simulink model "attitude_control"  (R2018a)
settings: Solver=VariableStepAuto  StartTime=0.0  StopTime=20  RelTol=1e-3
undefined symbols (not defined in the file): drone, matrix_A, matrix_B, matrix_C, matrix_D, obs_L, reg_K, simulation_sampling_ts
libraries: simulink x1
settings Model: Creator=ros  LastModifiedBy=ros

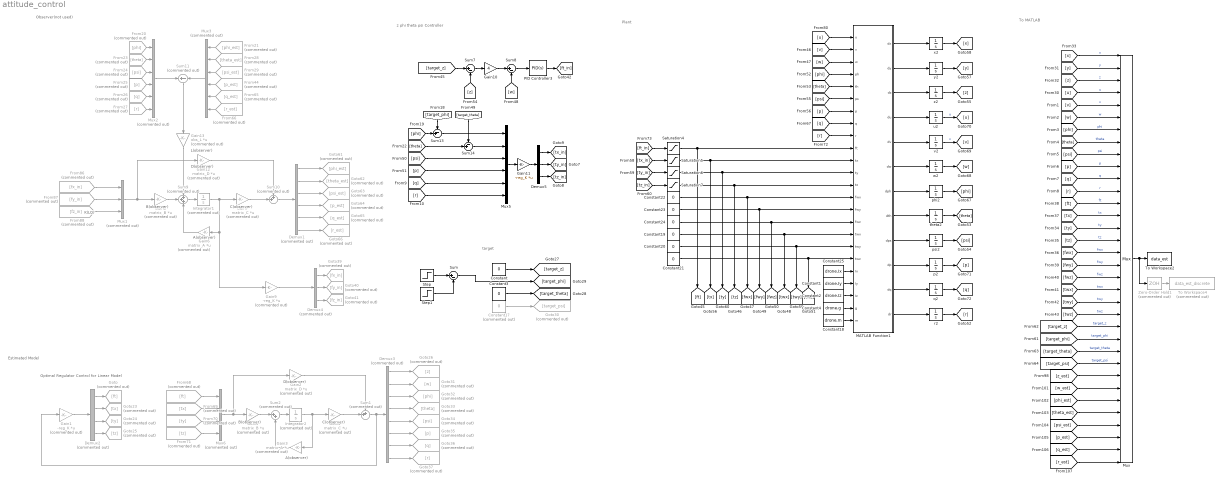
== system attitude_control ==
  note: B(observer)
  note: C(observer)
  note: A(observer)
  note: D(observer)
  note: L(observer)
  note: Optimal Regulator Control for Linear Model
  note: D(observer)
  note: C(observer)
  note: A(observer)
  note: B(observer)
  note: K(LQ)
  note: Plant
  note: To MATLAB
  note: target
  note: Estimated Model
  note: Observer(not used)
  note: z phi theta psi Controller
  Constant{,3,19..24} (8 alike) : Constant  Value=0
  Constant1 : Constant  Value=drone.Iy
  Constant17 : Constant  Commented=on  Value=0
  Constant18 : Constant  Value=drone.m
  Constant2 : Constant  Value=drone.Iz
  Constant25 : Constant  Value=drone.Ix
  Constant4 : Constant  Value=drone.g
  Demux1 : Demux  Commented=on  Outputs=6
  Demux2 : Demux  Commented=on
  Demux3 : Demux  Commented=on  Outputs=8
  Demux4 : Demux  Commented=on  Outputs=3
  Demux5 : Demux  Outputs=3
  From20 : From  Commented=on  GotoTag=phi
  From21 : From  Commented=on  GotoTag=phi_est
  From23 : From  Commented=on  GotoTag=theta
  From24 : From  Commented=on  GotoTag=psi
  From25 : From  Commented=on  GotoTag=p
  From26 : From  Commented=on  GotoTag=q
  From27 : From  Commented=on  GotoTag=r
  From28 : From  Commented=on  GotoTag=theta_est
  From29 : From  Commented=on  GotoTag=psi_est
  From44 : From  Commented=on  GotoTag=p_est
  From65 : From  Commented=on  GotoTag=q_est
  From66 : From  Commented=on  GotoTag=r_est
  From68 : From  Commented=on  GotoTag=ft
  From69 : From  Commented=on  GotoTag=tx
  From70 : From  Commented=on  GotoTag=ty
  From71 : From  Commented=on  GotoTag=tz
  From86 : From  Commented=on  GotoTag=fx_in
  From87 : From  Commented=on  GotoTag=fy_in
  From88 : From  Commented=on  GotoTag=fz_in
  Gain1 : Gain  Commented=on  Gain=-reg_K  Multiplication=Matrix(K*u)
  Gain10 : Gain  Gain=4
  Gain11 : Gain  Gain=-reg_K  Multiplication=Matrix(K*u)
  Gain12 : Gain  Commented=on  Gain=matrix_D  Multiplication=Matrix(K*u)
  Gain13 : Gain  Commented=on  Gain=obs_L  Multiplication=Matrix(K*u)
  Gain2 : Gain  Commented=on  Gain=matrix_D  Multiplication=Matrix(K*u)
  Gain3 : Gain  Commented=on  Gain=matrix_A  Multiplication=Matrix(K*u)
  Gain4 : Gain  Commented=on  Gain=matrix_C  Multiplication=Matrix(K*u)
  Gain5 : Gain  Commented=on  Gain=matrix_B  Multiplication=Matrix(K*u)
  Gain6 : Gain  Commented=on  Gain=matrix_A  Multiplication=Matrix(K*u)
  Gain7 : Gain  Commented=on  Gain=matrix_C  Multiplication=Matrix(K*u)
  Gain8 : Gain  Commented=on  Gain=matrix_B  Multiplication=Matrix(K*u)
  Gain9 : Gain  Commented=on  Gain=-reg_K  Multiplication=Matrix(K*u)
  Goto : Goto  Commented=on  GotoTag=ft
  Goto23 : Goto  Commented=on  GotoTag=tx
  Goto24 : Goto  Commented=on  GotoTag=ty
  Goto25 : Goto  Commented=on  GotoTag=tz
  Goto26 : Goto  Commented=on  GotoTag=z
  Goto30 : Goto  Commented=on  GotoTag=target_psi
  Goto31 : Goto  Commented=on  GotoTag=w
  Goto32 : Goto  Commented=on  GotoTag=phi
  Goto33 : Goto  Commented=on  GotoTag=theta
  Goto34 : Goto  Commented=on  GotoTag=psi
  Goto35 : Goto  Commented=on  GotoTag=p
  Goto36 : Goto  Commented=on  GotoTag=q
  Goto37 : Goto  Commented=on  GotoTag=r
  Goto39 : Goto  Commented=on  GotoTag=fx_in
  Goto40 : Goto  Commented=on  GotoTag=fy_in
  Goto41 : Goto  Commented=on  GotoTag=fz_in
  Goto61 : Goto  Commented=on  GotoTag=phi_est
  Goto62 : Goto  Commented=on  GotoTag=theta_est
  Goto63 : Goto  Commented=on  GotoTag=psi_est
  Goto64 : Goto  Commented=on  GotoTag=p_est
  Goto65 : Goto  Commented=on  GotoTag=q_est
  Goto66 : Goto  Commented=on  GotoTag=r_est
  Integrator1 : Integrator  Commented=on  InitialCondition=[0 0 0 0 0 0 0 0]
  Integrator2 : Integrator  Commented=on  InitialCondition=[-5 0 0 0 0 0 0 0]
  MATLAB Function1 : MATLAB Function  TreatAsAtomicUnit=on
  Mux : Mux  Inputs=34
      settings: DisplayOption=signals
  Mux1 : Mux  Commented=on  Inputs=3
  Mux2 : Mux  Commented=on  Inputs=6
  Mux3 : Mux  Commented=on  Inputs=6
  Mux5 : Mux  Inputs=6
  Mux6 : Mux  Commented=on
  PID Controller3 : simulink/Continuous/PID Controller  Controller=PID  TimeDomain=Continuous-time  SampleTime=-1  IntegratorMethod=Forward Euler  FilterMethod=Forward Euler  Form=Parallel  UseFilter=on  ControllerParametersSource=internal  P=7  I=6  D=0.7  N=100  InitialConditionSource=internal  InitialConditionForIntegrator=0  InitialConditionForFilter=0  ExternalReset=none  LimitOutput=off  UpperSaturationLimit=inf  LowerSaturationLimit=-inf  LinearizeAsGain=on  AntiWindupMode=none  Kb=1  TrackingMode=off  Kt=1  PParamMin=[]  PParamMax=[]  IParamMin=[]  IParamMax=[]  DParamMin=[]  DParamMax=[]  NParamMin=[]  NParamMax=[]  KbParamMin=[]  KbParamMax=[]  KtParamMin=[]  KtParamMax=[]  POutMin=[]  POutMax=[]  IOutMin=[]  IOutMax=[]  DOutMin=[]  DOutMax=[]  NOutMin=[]  NOutMax=[]  KbOutMin=[]  KbOutMax=[]  KtOutMin=[]  KtOutMax=[]  IntegratorOutMin=[]  IntegratorOutMax=[]  FilterOutMin=[]  FilterOutMax=[]  SumOutMin=[]  SumOutMax=[]  SumI1OutMin=[]  SumI1OutMax=[]  SumI2OutMin=[]  SumI2OutMax=[]  SumI3OutMin=[]  SumI3OutMax=[]  SumDOutMin=[]  SumDOutMax=[]  SaturationOutMin=[]  SaturationOutMax=[]  IntegratorContinuousStateAttributes=''  IntegratorStateMustResolveToSignalObject=off  IntegratorRTWStateStorageClass=Auto  FilterContinuousStateAttributes=''  FilterStateMustResolveToSignalObject=off  FilterRTWStateStorageClass=Auto  DifferentiatorICPrevScaledInput=0  DifferentiatorOutMin=[]  DifferentiatorOutMax=[]  FilterDiffOutCoefMin=[]  FilterDiffOutCoefMax=[]  SumDenOutMin=[]  SumDenOutMax=[]  SumNumOutMin=[]  SumNumOutMax=[]  ReciprocalOutMin=[]  ReciprocalOutMax=[]  DivideOutMin=[]  DivideOutMax=[]  TunerSelectOption=Transfer Function Based (PID Tuner App)
  Saturation{4..7} (4 alike) : Saturate  UpperLimit=30  LowerLimit=-100
  Step : Step  After=5*pi/180  SampleTime=0
  Step1 : Step  Time=6  After=5*pi/180  SampleTime=0
  Sum : Sum  Inputs=|+-
  Sum1 : Sum  Commented=on  Inputs=++|
  Sum10 : Sum  Commented=on  Inputs=++|
  Sum11 : Sum  Commented=on  Inputs=+-
  Sum13 : Sum  Inputs=-+|
  Sum14 : Sum  Inputs=-+|
  Sum2 : Sum  Commented=on  Inputs=|++
  Sum7 : Sum  Inputs=|+-
  Sum8 : Sum  Inputs=|+-
  Sum9 : Sum  Commented=on  Inputs=+++
  To Workspace2 : ToWorkspace  VariableName=data_est  SaveFormat=Timeseries  SampleTime=-1
  To Workspace4 : ToWorkspace  Commented=on  VariableName=data_est_discrete  SaveFormat=Timeseries  SampleTime=-1
  Zero-Order Hold1 : ZeroOrderHold  Commented=on  SampleTime=simulation_sampling_ts
  p2 : Integrator
  phi2 : Integrator
  psi2 : Integrator
  q2 : Integrator
  r2 : Integrator
  theta2 : Integrator
  u2 : Integrator
  v2 : Integrator
  w2 : Integrator
  x2 : Integrator
  y2 : Integrator
  z2 : Integrator
  wires:
  [x] -> Mux/1  "x"
  [v] -> Mux/5  "v"
  [z] -> Mux/3  "z"
  [w] -> Mux/6  "w"
  [p] -> Mux/10  "p"
  [phi] -> Mux/7  "phi"
  [theta] -> Mux/8  "theta"
  [r] -> Mux/12  "r"
  [y] -> Mux/2  "y"
  [psi] -> Mux/9  "psi"
  [u] -> Mux/4  "u"
  [q] -> Mux/11  "q"
  Mux/1 -> Zero-Order Hold1/1, To Workspace2/1
  [ft] -> Mux/13  "ft"
  [tx] -> Mux/14  "tx"
  [ty] -> Mux/15  "ty"
  [tz] -> Mux/16  "tz"
  [fwx] -> Mux/17  "fwx"
  [fwy] -> Mux/18  "fwy"
  [fwz] -> Mux/19  "fwz"
  [twx] -> Mux/20  "twx"
  [twy] -> Mux/21  "twy"
  [twz] -> Mux/22  "twz"
  Zero-Order Hold1/1 -> To Workspace4/1
  [target_z] -> Mux/23  "target_z"
  [target_phi] -> Mux/24  "target_phi"
  [target_theta] -> Mux/25  "target_theta"
  [target_psi] -> Mux/26  "target_psi"
  Constant17/1 -> Goto30/1
  Constant/1 -> [target_z]
  Sum/1 -> [target_phi]
  Mux1/1 -> Gain12/1, Gain8/1
  Sum9/1 -> Integrator1/1
  Integrator1/1 -> Gain7/1, Gain9/1, Gain6/1
  Gain8/1 -> Sum9/2
  Gain6/1 -> Sum9/3
  Gain7/1 -> Sum10/2
  Gain12/1 -> Sum10/1
  Sum10/1 -> Demux1/1
  Gain13/1 -> Sum9/1
  Mux3/1 -> Sum11/2
  Mux2/1 -> Sum11/1
  Sum11/1 -> Gain13/1
  [z_est] -> Mux/27
  [w_est] -> Mux/28
  [phi_est] -> Mux/29
  [theta_est] -> Mux/30
  [psi_est] -> Mux/31
  [p_est] -> Mux/32
  [q_est] -> Mux/33
  [r_est] -> Mux/34
  Demux2/3 -> Goto24/1
  Demux2/2 -> Goto23/1
  Demux2/4 -> Goto25/1
  Gain1/1 -> Demux2/1
  Demux2/1 -> Goto/1
  Gain4/1 -> Sum1/2
  Demux3/2 -> Goto31/1
  Demux3/1 -> Goto26/1
  Demux3/4 -> Goto33/1
  Gain2/1 -> Sum1/1
  Sum1/1 -> Gain1/1, Demux3/1
  Demux3/5 -> Goto34/1
  Demux3/8 -> Goto37/1
  Demux3/7 -> Goto36/1
  Sum2/1 -> Integrator2/1
  Demux3/6 -> Goto35/1
  Demux3/3 -> Goto32/1
  Gain3/1 -> Sum2/2
  Gain5/1 -> Sum2/1
  Integrator2/1 -> Gain4/1, Gain3/1
  Gain9/1 -> Demux4/1
  From69/1 -> Mux6/2
  From71/1 -> Mux6/4
  From70/1 -> Mux6/3
  From68/1 -> Mux6/1
  Mux6/1 -> Gain2/1, Gain5/1
  Gain10/1 -> Sum8/1
  Sum8/1 -> PID Controller3/1
  PID Controller3/1 -> [ft_in]
  [target_z] -> Sum7/1
  [z] -> Sum7/2
  Sum7/1 -> Gain10/1
  [w] -> Sum8/2
  Demux4/1 -> Goto39/1
  Demux4/2 -> Goto40/1
  Demux4/3 -> Goto41/1
  Demux1/1 -> Goto61/1
  Demux1/2 -> Goto62/1
  Demux1/4 -> Goto64/1
  Demux1/3 -> Goto63/1
  Demux1/6 -> Goto66/1
  Demux1/5 -> Goto65/1
  From88/1 -> Mux1/3
  From86/1 -> Mux1/1
  From87/1 -> Mux1/2
  From29/1 -> Mux3/3
  From44/1 -> Mux3/4
  From66/1 -> Mux3/6
  From65/1 -> Mux3/5
  From21/1 -> Mux3/1
  From28/1 -> Mux3/2
  From24/1 -> Mux2/3
  From27/1 -> Mux2/6
  From20/1 -> Mux2/1
  From26/1 -> Mux2/5
  From23/1 -> Mux2/2
  From25/1 -> Mux2/4
  u2/1 -> [u]  "u"
  Saturation4/1 -> [ft], MATLAB Function1/10(ft)
  phi2/1 -> [phi]
  y2/1 -> [y]
  Saturation7/1 -> [tz], MATLAB Function1/13(tz)
  v2/1 -> [v]  "v"
  MATLAB Function1/2(dy) -> y2/1
  [psi] -> MATLAB Function1/6(ps)
  [ty_in] -> Saturation6/1
  Constant2/1 -> MATLAB Function1/22(Iz)
  Constant19/1 -> [twx], MATLAB Function1/17(twx)
  MATLAB Function1/6(dw) -> w2/1
  r2/1 -> [r]
  Constant25/1 -> MATLAB Function1/20(Ix)
  MATLAB Function1/9(dps) -> psi2/1
  [p] -> MATLAB Function1/7(p)
  Constant1/1 -> MATLAB Function1/21(Iy)
  psi2/1 -> [psi]
  Constant20/1 -> [twy], MATLAB Function1/18(twy)
  MATLAB Function1/8(dth) -> theta2/1
  x2/1 -> [x]
  MATLAB Function1/3(dz) -> z2/1
  [tz_in] -> Saturation7/1
  MATLAB Function1/5(dv) -> v2/1
  MATLAB Function1/1(dx) -> x2/1
  z2/1 -> [z]
  MATLAB Function1/10(dp) -> p2/1
  q2/1 -> [q]
  Constant21/1 -> [twz], MATLAB Function1/19(twz)
  MATLAB Function1/11(dq) -> q2/1
  w2/1 -> [w]
  [theta] -> MATLAB Function1/5(th)
  Constant22/1 -> [fwx], MATLAB Function1/14(fwx)
  Constant4/1 -> MATLAB Function1/23(g)
  Saturation6/1 -> [ty], MATLAB Function1/12(ty)
  [q] -> MATLAB Function1/8(q)
  Constant24/1 -> [fwz], MATLAB Function1/16(fwz)
  theta2/1 -> [theta]
  [tx_in] -> Saturation5/1
  MATLAB Function1/4(du) -> u2/1
  Saturation5/1 -> [tx], MATLAB Function1/11(tx)
  [u] -> MATLAB Function1/1(u)
  MATLAB Function1/12(dr) -> r2/1
  [phi] -> MATLAB Function1/4(ph)
  Constant23/1 -> [fwy], MATLAB Function1/15(fwy)
  MATLAB Function1/7(dph) -> phi2/1
  Constant18/1 -> MATLAB Function1/24(m)
  [r] -> MATLAB Function1/9(r)
  [ft_in] -> Saturation4/1
  p2/1 -> [p]
  [w] -> MATLAB Function1/3(w)
  [v] -> MATLAB Function1/2(v)
  Demux5/3 -> [tz_in]
  [p] -> Mux5/4
  Mux5/1 -> Gain11/1
  Demux5/1 -> [tx_in]
  [q] -> Mux5/5
  [theta] -> Sum14/2
  Gain11/1 -> Demux5/1
  [target_phi] -> Sum13/1
  [r] -> Mux5/6
  [target_theta] -> Sum14/1
  Sum13/1 -> Mux5/1
  Sum14/1 -> Mux5/2
  [psi] -> Mux5/3
  [phi] -> Sum13/2
  Demux5/2 -> [ty_in]
  Step/1 -> Sum/1
  Step1/1 -> Sum/2
  Constant3/1 -> [target_theta]

== matlab function attitude_control/MATLAB Function1 ==
  data: u input; v input; dx output; w input; ph input; th input; ps input; p input; q input; r input; ft input; tx input; ty input; tz input; fwx input; fwy input; fwz input; twx input; twy input; twz input; dy output; dz output; du output; dv output; dw output; dph output; dth output; dps output; dp output; dq output; dr output; Ix input; Iy input; Iz input; g input; m input
function [dx, dy, dz, du, dv, dw, dph, dth, dps, dp, dq, dr] = fcn(u, v, w, ph, th, ps, p, q, r, ft, tx, ty, tz, fwx, fwy, fwz, twx, twy, twz, Ix, Iy, Iz, g, m)

dx = w*(sin(ph)*sin(ps) + cos(ph)*cos(ps)*sin(th)) - v*(cos(ph)*sin(ps) - cos(ps)*sin(ph)*sin(th)) + u*(cos(ps)*cos(th));
dy = v*(cos(ph)*cos(ps) + sin(ph)*sin(ps)*sin(th)) - w*(cos(ps)*sin(ph) - cos(ph)*sin(ps)*sin(th)) + u*(cos(th)*sin(ps));
dz = w*(cos(ph)*cos(th)) - u*(sin(th)) + v*(cos(th)*sin(ph));
du = r*v - q*w + g*(sin(th)) + fwx / m;
dv = p*w - r*u - g*(sin(ph)*cos(th)) + fwy / m;
dw = q*u - p*v - g*(cos(th)*cos(ph)) + (fwz + ft) / m;
dph = p + r*(cos(ph)*tan(th)) + q*(sin(ph)*tan(th));
dth = q*(cos(th)) - r*(sin(ph));
dps = r*(cos(ph)/cos(th)) + q*(sin(ph)/cos(th));
dp = r*q*(Iy - Iz)/Ix + (tx + twx)/Ix;
dq = p*r*(Iz - Ix)/Iy + (ty + twy)/Iy;
dr = p*q*(Ix - Iy)/Iz + (tz + twz)/Iz;
